simulink model "ASM_Traffic_V2X_Complete_Model_2"  (R2019a)
settings: Solver=ode1  StartTime=SIM.tstart.v  StopTime=Inf  FixedStep=SIM.StepSize.v  RelTol=1e-3
PostLoadFcn:
  | if any(exist('dsrtsu_mdlpostloadfcn', 'file') ~= 0), dsrtsu_mdlpostloadfcn('Execute', bdroot); end
  | try, asm_mdl_postloadfcn(bdroot, 'UpdateModel', 2200); catch, disp(lasterr); end,
undefined symbols (not defined in the file): _SensorPnts_1, _SensorPnts_13, _SensorPnts_17, _SensorPnts_21, _SensorPnts_25, _SensorPnts_29, _SensorPnts_33, _SensorPnts_37, _SensorPnts_41, _SensorPnts_45, _SensorPnts_49, _SensorPnts_5, _SensorPnts_53, _SensorPnts_57, _SensorPnts_9, _to_, CPT, G5A, ITS, MDL, rad, s_to_rpm, SIM
libraries: simulink x169, ASM_VehicleDynamics_lib x126, ASM_Traffic_lib x83, ASM_Utils_lib x49, mdbs x45, ASM_Environment_lib x17, dspindex x12, dsaV2xLibraryAux x10, dsmpblib x6, dsaV2xAsn1Library x4, dsaV2xLibrary x4, ASM_BrakeHydraulics_lib x4
(part 14 of 36)

== system ASM_Traffic_V2X_Complete_Model_2/MDL/VehicleDynamics/Tire/Tire_FR ==
  Coeff_Fric_Road[] : Inport
  " Pos_z_CP_CoorSys_E[m]" : Inport  Port=2
  UnitVec_z_CP_CoorSys_E[x;y;z] : Inport  Port=3
  Pos_Wheels_CoorSys_E[x;y;z][m] : Inport  Port=4
  v_WheelBody_Abs_CoorSys_V[x;y;z][m|s] : Inport  Port=5
  w_Wheel_CoorSys_Abs_V[x;y;z][rad|s] : Inport  Port=6
  RotationMatrix_V_E_T[3x3] : Inport  Port=7
  UnitVec_y_Wheel_CoorSys_V[x;y;z] : Inport  Port=8
  omega_Wheel[rad|s] : Inport  Port=9
  Sw_Tire_Parameter_Set[1|2|3|4] : Inport  Port=10
  Sw_Tire_Model[1TMEasy|2MF] : Inport  Port=11
  Reset[] : Inport  Port=12
  Mode[1Normal|2Mirror] : Inport  Port=13
  p[Pa] : Inport  Port=14
  Bus Selector : BusSelector  OutputSignals=Sw_r_Tire[1:intern;2:extern],r_Tire_extern[m]
  CONTACT_POINT_CALCULATION_FR : ASM_VehicleDynamics_lib/VehicleDynamics/Tire/Tire_FR/CONTACT_POINT_CALCULATION_FR  Tag=ASM_SUBCOMPONENT  ASMProperties=struct('Name','CONTACT_POINT_CALCULATION_FR','Version','6.0','Library','ASM_VehicleDynamics_lib')  ASMInstanceName=contact_point_calculation_fr  ASMInstanceID=1
  Compare To Constant : simulink/Logic and Bit Operations/Compare To Constant  relop===  const=1  OutDataTypeStr=boolean  ZeroCross=off
  Demux : Demux  Outputs=[1 1 1 1 1 1 1]
  EnableMF : simulink/Logic and Bit Operations/Compare To Constant  relop=~=  const=2  OutDataTypeStr=boolean  ZeroCross=off
  IncludedInASMBUS : Terminator
  Multiport Switch : MultiPortSwitch  Inputs=2  SaturateOnIntegerOverflow=on
  Mux : Mux  Inputs=7
  Or : Logic  Operator=OR  AllPortsSameDT=off  OutDataTypeStr=boolean
  TIRE_FORCES_AND_TORQUES_VECTORS_FR : ASM_VehicleDynamics_lib/VehicleDynamics/Tire/Tire_FR/TIRE_FORCES_AND_TORQUES_VECTORS_FR  Tag=ASM_SUBCOMPONENT  ASMProperties=struct('Name','TIRE_FORCES_AND_TORQUES_VECTORS_FR','Version','1.0','Library','ASM_VehicleDynamics_lib')  ASMInstanceName=tire_forces_and_torques_vectors_fr  ASMInstanceID=1
  TIRE_MF : ASM_VehicleDynamics_lib/VehicleDynamics/Tire/TireComponents/TIRE_MF  Tag=ASM_SUBCOMPONENT  Base=MDL.VehicleDynamics.Tire.FR.MF.Base  Para_Set_1=MDL.VehicleDynamics.Tire.FR.MF.Para_Set_1  Para_Set_2=MDL.VehicleDynamics.Tire.FR.MF.Para_Set_2  Para_Set_3=MDL.VehicleDynamics.Tire.FR.MF.Para_Set_3  Para_Set_4=MDL.VehicleDynamics.Tire.FR.MF.Para_Set_4  StepSize=SIM.StepSize  ASMProperties=struct('Name','TIRE_MF','Version','4.0','Library','ASM_VehicleDynamics_lib')  ASMInstanceName=FR  ASMInstanceID=2
      settings: AttributesFormatString=Instance Name: FR\nInstance ID: 2
  TIRE_MODEL_TMEASY_FR : ASM_VehicleDynamics_lib/VehicleDynamics/Tire/Tire_FR/TIRE_MODEL_TMEASY_FR  Tag=ASM_SUBCOMPONENT  Para_Set_1=MDL.VehicleDynamics.Tire.FR.TMEasy.Para_Set_1  Para_Set_2=MDL.VehicleDynamics.Tire.FR.TMEasy.Para_Set_2  Para_Set_3=MDL.VehicleDynamics.Tire.FR.TMEasy.Para_Set_3  Para_Set_4=MDL.VehicleDynamics.Tire.FR.TMEasy.Para_Set_4  StepSize=SIM.StepSize  ASMProperties=struct('Name','TIRE_MODEL_TMEASY_FR','Version','16.0','Library','ASM_VehicleDynamics_lib')  ASMInstanceName=tire_model_tmeasy_fr  ASMInstanceID=1
  F_Tire[x;y;z][N] : Outport
  Trq_Tire[x;y;z][Nm] : Outport  Port=2
  Trq_Tire_Wheel[Nm] : Outport  Port=3
  Stiffness_z_Tire[N|m] : Outport  Port=4
  tag scope: ASMBUS_VehicleDynamics_ContactPoint_FR_Tire=global, ASMBUS_VehicleDynamics_ForcesAndTorques_FR_Tire=global, ASMBUS_VehicleDynamics_MF_FR_Tire=global, ASMBUS_VehicleDynamics_TMEasy_FR_Tire=global
  wires:
  p[Pa]/1 -> TIRE_MF/13
  Mode[1Normal|2Mirror]/1 -> TIRE_MF/12
  Or/1 -> TIRE_MF/9
  EnableMF/1 -> Or/1
  TIRE_MF/2 -> Multiport Switch/3
  Bus Selector/1 -> TIRE_MODEL_TMEASY_FR/10, TIRE_MF/10  "<Sw_r_Tire[1:intern;2:extern]>"
  Bus Selector/2 -> TIRE_MODEL_TMEASY_FR/11, TIRE_MF/11  "<r_Tire_extern[m]>"
  [TAG_Tire_Switches] -> Bus Selector/1
  Multiport Switch/1 -> Demux/1
  Demux/6 -> TIRE_FORCES_AND_TORQUES_VECTORS_FR/6
  Demux/5 -> TIRE_FORCES_AND_TORQUES_VECTORS_FR/5
  Demux/4 -> TIRE_FORCES_AND_TORQUES_VECTORS_FR/4
  Demux/3 -> TIRE_FORCES_AND_TORQUES_VECTORS_FR/3
  Demux/2 -> TIRE_FORCES_AND_TORQUES_VECTORS_FR/2
  Demux/1 -> TIRE_FORCES_AND_TORQUES_VECTORS_FR/1
  Demux/7 -> Stiffness_z_Tire[N|m]/1
  Mux/1 -> Multiport Switch/2
  TIRE_MODEL_TMEASY_FR/8 -> Mux/7
  TIRE_MODEL_TMEASY_FR/7 -> Mux/6
  TIRE_MODEL_TMEASY_FR/6 -> Mux/5
  TIRE_MODEL_TMEASY_FR/5 -> Mux/4
  TIRE_MODEL_TMEASY_FR/4 -> Mux/3
  TIRE_MODEL_TMEASY_FR/3 -> Mux/2
  TIRE_MODEL_TMEASY_FR/2 -> Mux/1
  Reset[]/1 -> Or/2, TIRE_MODEL_TMEASY_FR/9, CONTACT_POINT_CALCULATION_FR/8
  CONTACT_POINT_CALCULATION_FR/11 -> IncludedInASMBUS/1
  CONTACT_POINT_CALCULATION_FR/1 -> [ASMBUS_VehicleDynamics_ContactPoint_FR_Tire]
  TIRE_MF/1 -> [ASMBUS_VehicleDynamics_MF_FR_Tire]
  TIRE_MODEL_TMEASY_FR/1 -> [ASMBUS_VehicleDynamics_TMEasy_FR_Tire]
  Compare To Constant/1 -> TIRE_MODEL_TMEASY_FR/Enable
  RotationMatrix_V_E_T[3x3]/1 -> CONTACT_POINT_CALCULATION_FR/6
  UnitVec_z_CP_CoorSys_E[x;y;z]/1 -> CONTACT_POINT_CALCULATION_FR/5
  " Pos_z_CP_CoorSys_E[m]"/1 -> CONTACT_POINT_CALCULATION_FR/4
  Pos_Wheels_CoorSys_E[x;y;z][m]/1 -> CONTACT_POINT_CALCULATION_FR/3
  w_Wheel_CoorSys_Abs_V[x;y;z][rad|s]/1 -> CONTACT_POINT_CALCULATION_FR/2
  v_WheelBody_Abs_CoorSys_V[x;y;z][m|s]/1 -> CONTACT_POINT_CALCULATION_FR/1
  Sw_Tire_Parameter_Set[1|2|3|4]/1 -> TIRE_MODEL_TMEASY_FR/1, TIRE_MF/1
  TIRE_FORCES_AND_TORQUES_VECTORS_FR/1 -> [ASMBUS_VehicleDynamics_ForcesAndTorques_FR_Tire]
  Coeff_Fric_Road[]/1 -> TIRE_MODEL_TMEASY_FR/2, TIRE_MF/2
  omega_Wheel[rad|s]/1 -> TIRE_MODEL_TMEASY_FR/3, TIRE_MF/3
  UnitVec_y_Wheel_CoorSys_V[x;y;z]/1 -> TIRE_FORCES_AND_TORQUES_VECTORS_FR/11, CONTACT_POINT_CALCULATION_FR/7
  CONTACT_POINT_CALCULATION_FR/2 -> TIRE_MODEL_TMEASY_FR/4, TIRE_MF/4
  CONTACT_POINT_CALCULATION_FR/3 -> TIRE_MODEL_TMEASY_FR/5, TIRE_MF/5
  CONTACT_POINT_CALCULATION_FR/4 -> TIRE_MODEL_TMEASY_FR/6, TIRE_MF/6
  CONTACT_POINT_CALCULATION_FR/5 -> TIRE_MODEL_TMEASY_FR/7, TIRE_MF/7
  CONTACT_POINT_CALCULATION_FR/6 -> TIRE_MODEL_TMEASY_FR/8, TIRE_MF/8
  TIRE_FORCES_AND_TORQUES_VECTORS_FR/2 -> F_Tire[x;y;z][N]/1
  TIRE_FORCES_AND_TORQUES_VECTORS_FR/4 -> Trq_Tire_Wheel[Nm]/1
  TIRE_FORCES_AND_TORQUES_VECTORS_FR/3 -> Trq_Tire[x;y;z][Nm]/1
  CONTACT_POINT_CALCULATION_FR/7 -> TIRE_FORCES_AND_TORQUES_VECTORS_FR/7
  CONTACT_POINT_CALCULATION_FR/8 -> TIRE_FORCES_AND_TORQUES_VECTORS_FR/8
  CONTACT_POINT_CALCULATION_FR/9 -> TIRE_FORCES_AND_TORQUES_VECTORS_FR/9
  CONTACT_POINT_CALCULATION_FR/10 -> TIRE_FORCES_AND_TORQUES_VECTORS_FR/10
  Sw_Tire_Model[1TMEasy|2MF]/1 -> Compare To Constant/1, Multiport Switch/1, EnableMF/1

== system ASM_Traffic_V2X_Complete_Model_2/MDL/VehicleDynamics/Tire/Tire_RL ==
  Coeff_Fric_Road[] : Inport
  " Pos_z_CP_CoorSys_E[m]" : Inport  Port=2
  UnitVec_z_CP_CoorSys_E[x;y;z] : Inport  Port=3
  Pos_Wheels_CoorSys_E[x;y;z][m] : Inport  Port=4
  v_WheelBody_Abs_CoorSys_V[x;y;z][m|s] : Inport  Port=5
  w_Wheel_CoorSys_Abs_V[x;y;z][rad|s] : Inport  Port=6
  RotationMatrix_V_E_T[3x3] : Inport  Port=7
  UnitVec_y_Wheel_CoorSys_V[x;y;z] : Inport  Port=8
  omega_Wheel[rad|s] : Inport  Port=9
  Sw_Tire_Parameter_Set[1|2|3|4] : Inport  Port=10
  Sw_Tire_Model[1TMEasy|2MF] : Inport  Port=11
  Reset[] : Inport  Port=12
  Mode[1Normal|2Mirror] : Inport  Port=13
  p[Pa] : Inport  Port=14
  Bus Selector : BusSelector  OutputSignals=Sw_r_Tire[1:intern;2:extern],r_Tire_extern[m]
  CONTACT_POINT_CALCULATION_RL : ASM_VehicleDynamics_lib/VehicleDynamics/Tire/Tire_RL/CONTACT_POINT_CALCULATION_RL  Tag=ASM_SUBCOMPONENT  ASMProperties=struct('Name','CONTACT_POINT_CALCULATION_RL','Version','6.0','Library','ASM_VehicleDynamics_lib')  ASMInstanceName=contact_point_calculation_rl  ASMInstanceID=1
  Compare To Constant : simulink/Logic and Bit Operations/Compare To Constant  relop===  const=1  OutDataTypeStr=boolean  ZeroCross=off
  Demux : Demux  Outputs=[1 1 1 1 1 1 1]
  EnableMF : simulink/Logic and Bit Operations/Compare To Constant  relop=~=  const=2  OutDataTypeStr=boolean  ZeroCross=off
  IncludedInASMBUS : Terminator
  Multiport Switch : MultiPortSwitch  Inputs=2  SaturateOnIntegerOverflow=on
  Mux : Mux  Inputs=7
  Or : Logic  Operator=OR  AllPortsSameDT=off  OutDataTypeStr=boolean
  TIRE_FORCES_AND_TORQUES_VECTORS_RL : ASM_VehicleDynamics_lib/VehicleDynamics/Tire/Tire_RL/TIRE_FORCES_AND_TORQUES_VECTORS_RL  Tag=ASM_SUBCOMPONENT  ASMProperties=struct('Name','TIRE_FORCES_AND_TORQUES_VECTORS_RL','Version','1.0','Library','ASM_VehicleDynamics_lib')  ASMInstanceName=tire_forces_and_torques_vectors_rl  ASMInstanceID=1
  TIRE_MF : ASM_VehicleDynamics_lib/VehicleDynamics/Tire/TireComponents/TIRE_MF  Tag=ASM_SUBCOMPONENT  Base=MDL.VehicleDynamics.Tire.RL.MF.Base  Para_Set_1=MDL.VehicleDynamics.Tire.RL.MF.Para_Set_1  Para_Set_2=MDL.VehicleDynamics.Tire.RL.MF.Para_Set_2  Para_Set_3=MDL.VehicleDynamics.Tire.RL.MF.Para_Set_3  Para_Set_4=MDL.VehicleDynamics.Tire.RL.MF.Para_Set_4  StepSize=SIM.StepSize  ASMProperties=struct('Name','TIRE_MF','Version','4.0','Library','ASM_VehicleDynamics_lib')  ASMInstanceName=RL  ASMInstanceID=3
      settings: AttributesFormatString=Instance Name: RL\nInstance ID: 3
  TIRE_MODEL_TMEASY_RL : ASM_VehicleDynamics_lib/VehicleDynamics/Tire/Tire_RL/TIRE_MODEL_TMEASY_RL  Tag=ASM_SUBCOMPONENT  Para_Set_1=MDL.VehicleDynamics.Tire.RL.TMEasy.Para_Set_1  Para_Set_2=MDL.VehicleDynamics.Tire.RL.TMEasy.Para_Set_2  Para_Set_3=MDL.VehicleDynamics.Tire.RL.TMEasy.Para_Set_3  Para_Set_4=MDL.VehicleDynamics.Tire.RL.TMEasy.Para_Set_4  StepSize=SIM.StepSize  ASMProperties=struct('Name','TIRE_MODEL_TMEASY_RL','Version','16.0','Library','ASM_VehicleDynamics_lib')  ASMInstanceName=tire_model_tmeasy_rl  ASMInstanceID=1
  F_Tire[x;y;z][N] : Outport
  Trq_Tire[x;y;z][Nm] : Outport  Port=2
  Trq_Tire_Wheel[Nm] : Outport  Port=3
  Stiffness_z_Tire[N|m] : Outport  Port=4
  tag scope: ASMBUS_VehicleDynamics_ContactPoint_RL_Tire=global, ASMBUS_VehicleDynamics_ForcesAndTorques_RL_Tire=global, ASMBUS_VehicleDynamics_MF_RL_Tire=global, ASMBUS_VehicleDynamics_TMEasy_RL_Tire=global
  wires:
  p[Pa]/1 -> TIRE_MF/13
  Mode[1Normal|2Mirror]/1 -> TIRE_MF/12
  Or/1 -> TIRE_MF/9
  EnableMF/1 -> Or/1
  TIRE_MF/2 -> Multiport Switch/3
  Bus Selector/2 -> TIRE_MODEL_TMEASY_RL/11, TIRE_MF/11  "<r_Tire_extern[m]>"
  Bus Selector/1 -> TIRE_MODEL_TMEASY_RL/10, TIRE_MF/10  "<Sw_r_Tire[1:intern;2:extern]>"
  [TAG_Tire_Switches] -> Bus Selector/1
  Multiport Switch/1 -> Demux/1
  Demux/7 -> Stiffness_z_Tire[N|m]/1
  Demux/6 -> TIRE_FORCES_AND_TORQUES_VECTORS_RL/6
  Demux/5 -> TIRE_FORCES_AND_TORQUES_VECTORS_RL/5
  Demux/4 -> TIRE_FORCES_AND_TORQUES_VECTORS_RL/4
  Demux/3 -> TIRE_FORCES_AND_TORQUES_VECTORS_RL/3
  Demux/2 -> TIRE_FORCES_AND_TORQUES_VECTORS_RL/2
  Demux/1 -> TIRE_FORCES_AND_TORQUES_VECTORS_RL/1
  Mux/1 -> Multiport Switch/2
  TIRE_MODEL_TMEASY_RL/8 -> Mux/7
  TIRE_MODEL_TMEASY_RL/7 -> Mux/6
  TIRE_MODEL_TMEASY_RL/6 -> Mux/5
  TIRE_MODEL_TMEASY_RL/5 -> Mux/4
  TIRE_MODEL_TMEASY_RL/4 -> Mux/3
  TIRE_MODEL_TMEASY_RL/3 -> Mux/2
  TIRE_MODEL_TMEASY_RL/2 -> Mux/1
  Reset[]/1 -> TIRE_MODEL_TMEASY_RL/9, Or/2, CONTACT_POINT_CALCULATION_RL/8
  CONTACT_POINT_CALCULATION_RL/11 -> IncludedInASMBUS/1
  TIRE_FORCES_AND_TORQUES_VECTORS_RL/1 -> [ASMBUS_VehicleDynamics_ForcesAndTorques_RL_Tire]
  CONTACT_POINT_CALCULATION_RL/1 -> [ASMBUS_VehicleDynamics_ContactPoint_RL_Tire]
  TIRE_MF/1 -> [ASMBUS_VehicleDynamics_MF_RL_Tire]
  TIRE_MODEL_TMEASY_RL/1 -> [ASMBUS_VehicleDynamics_TMEasy_RL_Tire]
  RotationMatrix_V_E_T[3x3]/1 -> CONTACT_POINT_CALCULATION_RL/6
  UnitVec_z_CP_CoorSys_E[x;y;z]/1 -> CONTACT_POINT_CALCULATION_RL/5
  " Pos_z_CP_CoorSys_E[m]"/1 -> CONTACT_POINT_CALCULATION_RL/4
  Pos_Wheels_CoorSys_E[x;y;z][m]/1 -> CONTACT_POINT_CALCULATION_RL/3
  w_Wheel_CoorSys_Abs_V[x;y;z][rad|s]/1 -> CONTACT_POINT_CALCULATION_RL/2
  v_WheelBody_Abs_CoorSys_V[x;y;z][m|s]/1 -> CONTACT_POINT_CALCULATION_RL/1
  Compare To Constant/1 -> TIRE_MODEL_TMEASY_RL/Enable
  Sw_Tire_Model[1TMEasy|2MF]/1 -> Compare To Constant/1, Multiport Switch/1, EnableMF/1
  CONTACT_POINT_CALCULATION_RL/10 -> TIRE_FORCES_AND_TORQUES_VECTORS_RL/10
  CONTACT_POINT_CALCULATION_RL/9 -> TIRE_FORCES_AND_TORQUES_VECTORS_RL/9
  CONTACT_POINT_CALCULATION_RL/8 -> TIRE_FORCES_AND_TORQUES_VECTORS_RL/8
  CONTACT_POINT_CALCULATION_RL/7 -> TIRE_FORCES_AND_TORQUES_VECTORS_RL/7
  TIRE_FORCES_AND_TORQUES_VECTORS_RL/3 -> Trq_Tire[x;y;z][Nm]/1
  TIRE_FORCES_AND_TORQUES_VECTORS_RL/4 -> Trq_Tire_Wheel[Nm]/1
  TIRE_FORCES_AND_TORQUES_VECTORS_RL/2 -> F_Tire[x;y;z][N]/1
  CONTACT_POINT_CALCULATION_RL/6 -> TIRE_MODEL_TMEASY_RL/8, TIRE_MF/8
  CONTACT_POINT_CALCULATION_RL/5 -> TIRE_MODEL_TMEASY_RL/7, TIRE_MF/7
  CONTACT_POINT_CALCULATION_RL/4 -> TIRE_MODEL_TMEASY_RL/6, TIRE_MF/6
  CONTACT_POINT_CALCULATION_RL/3 -> TIRE_MODEL_TMEASY_RL/5, TIRE_MF/5
  CONTACT_POINT_CALCULATION_RL/2 -> TIRE_MODEL_TMEASY_RL/4, TIRE_MF/4
  UnitVec_y_Wheel_CoorSys_V[x;y;z]/1 -> TIRE_FORCES_AND_TORQUES_VECTORS_RL/11, CONTACT_POINT_CALCULATION_RL/7
  omega_Wheel[rad|s]/1 -> TIRE_MODEL_TMEASY_RL/3, TIRE_MF/3
  Coeff_Fric_Road[]/1 -> TIRE_MODEL_TMEASY_RL/2, TIRE_MF/2
  Sw_Tire_Parameter_Set[1|2|3|4]/1 -> TIRE_MODEL_TMEASY_RL/1, TIRE_MF/1

== system ASM_Traffic_V2X_Complete_Model_2/MDL/VehicleDynamics/Tire/Tire_RR ==
  Coeff_Fric_Road[] : Inport
  " Pos_z_CP_CoorSys_E[m]" : Inport  Port=2
  UnitVec_z_CP_CoorSys_E[x;y;z] : Inport  Port=3
  Pos_Wheels_CoorSys_E[x;y;z][m] : Inport  Port=4
  v_WheelBody_Abs_CoorSys_V[x;y;z][m|s] : Inport  Port=5
  w_Wheel_CoorSys_Abs_V[x;y;z][rad|s] : Inport  Port=6
  RotationMatrix_V_E_T[3x3] : Inport  Port=7
  UnitVec_y_Wheel_CoorSys_V[x;y;z] : Inport  Port=8
  omega_Wheel[rad|s] : Inport  Port=9
  Sw_Tire_Parameter_Set[1|2|3|4] : Inport  Port=10
  Sw_Tire_Model[1TMEasy|2MF] : Inport  Port=11
  Reset[] : Inport  Port=12
  Mode[1Normal|2Mirror] : Inport  Port=13
  p[Pa] : Inport  Port=14
  Bus Selector : BusSelector  OutputSignals=Sw_r_Tire[1:intern;2:extern],r_Tire_extern[m]
  CONTACT_POINT_CALCULATION_RR : ASM_VehicleDynamics_lib/VehicleDynamics/Tire/Tire_RR/CONTACT_POINT_CALCULATION_RR  Tag=ASM_SUBCOMPONENT  ASMProperties=struct('Name','CONTACT_POINT_CALCULATION_RR','Version','6.0','Library','ASM_VehicleDynamics_lib')  ASMInstanceName=contact_point_calculation_rr  ASMInstanceID=1
  Compare To Constant : simulink/Logic and Bit Operations/Compare To Constant  relop===  const=1  OutDataTypeStr=boolean  ZeroCross=off
  Demux : Demux  Outputs=[1 1 1 1 1 1 1]
  EnableMF : simulink/Logic and Bit Operations/Compare To Constant  relop=~=  const=2  OutDataTypeStr=boolean  ZeroCross=off
  IncludedInASMBUS : Terminator
  Multiport Switch : MultiPortSwitch  Inputs=2  SaturateOnIntegerOverflow=on
  Mux : Mux  Inputs=7
  Or : Logic  Operator=OR  AllPortsSameDT=off  OutDataTypeStr=boolean
  TIRE_FORCES_AND_TORQUES_VECTORS_RR : ASM_VehicleDynamics_lib/VehicleDynamics/Tire/Tire_RR/TIRE_FORCES_AND_TORQUES_VECTORS_RR  Tag=ASM_SUBCOMPONENT  ASMProperties=struct('Name','TIRE_FORCES_AND_TORQUES_VECTORS_RR','Version','1.0','Library','ASM_VehicleDynamics_lib')  ASMInstanceName=tire_forces_and_torques_vectors_rr  ASMInstanceID=1
  TIRE_MF : ASM_VehicleDynamics_lib/VehicleDynamics/Tire/TireComponents/TIRE_MF  Tag=ASM_SUBCOMPONENT  Base=MDL.VehicleDynamics.Tire.RR.MF.Base  Para_Set_1=MDL.VehicleDynamics.Tire.RR.MF.Para_Set_1  Para_Set_2=MDL.VehicleDynamics.Tire.RR.MF.Para_Set_2  Para_Set_3=MDL.VehicleDynamics.Tire.RR.MF.Para_Set_3  Para_Set_4=MDL.VehicleDynamics.Tire.RR.MF.Para_Set_4  StepSize=SIM.StepSize  ASMProperties=struct('Name','TIRE_MF','Version','4.0','Library','ASM_VehicleDynamics_lib')  ASMInstanceName=RR  ASMInstanceID=4
      settings: AttributesFormatString=Instance Name: RR\nInstance ID: 4
  TIRE_MODEL_TMEASY_RR : ASM_VehicleDynamics_lib/VehicleDynamics/Tire/Tire_RR/TIRE_MODEL_TMEASY_RR  Tag=ASM_SUBCOMPONENT  Para_Set_1=MDL.VehicleDynamics.Tire.RR.TMEasy.Para_Set_1  Para_Set_2=MDL.VehicleDynamics.Tire.RR.TMEasy.Para_Set_2  Para_Set_3=MDL.VehicleDynamics.Tire.RR.TMEasy.Para_Set_3  Para_Set_4=MDL.VehicleDynamics.Tire.RR.TMEasy.Para_Set_4  StepSize=SIM.StepSize  ASMProperties=struct('Name','TIRE_MODEL_TMEASY_RR','Version','16.0','Library','ASM_VehicleDynamics_lib')  ASMInstanceName=tire_model_tmeasy_rr  ASMInstanceID=1
  F_Tire[x;y;z][N] : Outport
  Trq_Tire[x;y;z][Nm] : Outport  Port=2
  Trq_Tire_Wheel[Nm] : Outport  Port=3
  Stiffness_z_Tire[N|m] : Outport  Port=4
  tag scope: ASMBUS_VehicleDynamics_ContactPoint_RR_Tire=global, ASMBUS_VehicleDynamics_ForcesAndTorques_RR_Tire=global, ASMBUS_VehicleDynamics_MF_RR_Tire=global, ASMBUS_VehicleDynamics_TMEasy_RR_Tire=global
  wires:
  p[Pa]/1 -> TIRE_MF/13
  Mode[1Normal|2Mirror]/1 -> TIRE_MF/12
  Or/1 -> TIRE_MF/9
  EnableMF/1 -> Or/1
  TIRE_MF/2 -> Multiport Switch/3
  Bus Selector/2 -> TIRE_MODEL_TMEASY_RR/11, TIRE_MF/11  "<r_Tire_extern[m]>"
  Bus Selector/1 -> TIRE_MODEL_TMEASY_RR/10, TIRE_MF/10  "<Sw_r_Tire[1:intern;2:extern]>"
  [TAG_Tire_Switches] -> Bus Selector/1
  Multiport Switch/1 -> Demux/1
  Demux/7 -> Stiffness_z_Tire[N|m]/1
  Demux/6 -> TIRE_FORCES_AND_TORQUES_VECTORS_RR/6
  Demux/5 -> TIRE_FORCES_AND_TORQUES_VECTORS_RR/5
  Demux/4 -> TIRE_FORCES_AND_TORQUES_VECTORS_RR/4
  Demux/3 -> TIRE_FORCES_AND_TORQUES_VECTORS_RR/3
  Demux/2 -> TIRE_FORCES_AND_TORQUES_VECTORS_RR/2
  Demux/1 -> TIRE_FORCES_AND_TORQUES_VECTORS_RR/1
  Mux/1 -> Multiport Switch/2
  TIRE_MODEL_TMEASY_RR/8 -> Mux/7
  TIRE_MODEL_TMEASY_RR/7 -> Mux/6
  TIRE_MODEL_TMEASY_RR/6 -> Mux/5
  TIRE_MODEL_TMEASY_RR/5 -> Mux/4
  TIRE_MODEL_TMEASY_RR/4 -> Mux/3
  TIRE_MODEL_TMEASY_RR/3 -> Mux/2
  TIRE_MODEL_TMEASY_RR/2 -> Mux/1
  Reset[]/1 -> Or/2, TIRE_MODEL_TMEASY_RR/9, CONTACT_POINT_CALCULATION_RR/8
  CONTACT_POINT_CALCULATION_RR/11 -> IncludedInASMBUS/1
  TIRE_FORCES_AND_TORQUES_VECTORS_RR/1 -> [ASMBUS_VehicleDynamics_ForcesAndTorques_RR_Tire]
  CONTACT_POINT_CALCULATION_RR/1 -> [ASMBUS_VehicleDynamics_ContactPoint_RR_Tire]
  TIRE_MF/1 -> [ASMBUS_VehicleDynamics_MF_RR_Tire]
  TIRE_MODEL_TMEASY_RR/1 -> [ASMBUS_VehicleDynamics_TMEasy_RR_Tire]
  RotationMatrix_V_E_T[3x3]/1 -> CONTACT_POINT_CALCULATION_RR/6
  UnitVec_z_CP_CoorSys_E[x;y;z]/1 -> CONTACT_POINT_CALCULATION_RR/5
  " Pos_z_CP_CoorSys_E[m]"/1 -> CONTACT_POINT_CALCULATION_RR/4
  Pos_Wheels_CoorSys_E[x;y;z][m]/1 -> CONTACT_POINT_CALCULATION_RR/3
  w_Wheel_CoorSys_Abs_V[x;y;z][rad|s]/1 -> CONTACT_POINT_CALCULATION_RR/2
  v_WheelBody_Abs_CoorSys_V[x;y;z][m|s]/1 -> CONTACT_POINT_CALCULATION_RR/1
  Sw_Tire_Parameter_Set[1|2|3|4]/1 -> TIRE_MODEL_TMEASY_RR/1, TIRE_MF/1
  Coeff_Fric_Road[]/1 -> TIRE_MODEL_TMEASY_RR/2, TIRE_MF/2
  omega_Wheel[rad|s]/1 -> TIRE_MODEL_TMEASY_RR/3, TIRE_MF/3
  UnitVec_y_Wheel_CoorSys_V[x;y;z]/1 -> TIRE_FORCES_AND_TORQUES_VECTORS_RR/11, CONTACT_POINT_CALCULATION_RR/7
  CONTACT_POINT_CALCULATION_RR/2 -> TIRE_MODEL_TMEASY_RR/4, TIRE_MF/4
  CONTACT_POINT_CALCULATION_RR/3 -> TIRE_MODEL_TMEASY_RR/5, TIRE_MF/5
  CONTACT_POINT_CALCULATION_RR/4 -> TIRE_MODEL_TMEASY_RR/6, TIRE_MF/6
  CONTACT_POINT_CALCULATION_RR/5 -> TIRE_MODEL_TMEASY_RR/7, TIRE_MF/7
  CONTACT_POINT_CALCULATION_RR/6 -> TIRE_MODEL_TMEASY_RR/8, TIRE_MF/8
  TIRE_FORCES_AND_TORQUES_VECTORS_RR/2 -> F_Tire[x;y;z][N]/1
  TIRE_FORCES_AND_TORQUES_VECTORS_RR/4 -> Trq_Tire_Wheel[Nm]/1
  TIRE_FORCES_AND_TORQUES_VECTORS_RR/3 -> Trq_Tire[x;y;z][Nm]/1
  CONTACT_POINT_CALCULATION_RR/7 -> TIRE_FORCES_AND_TORQUES_VECTORS_RR/7
  CONTACT_POINT_CALCULATION_RR/8 -> TIRE_FORCES_AND_TORQUES_VECTORS_RR/8
  CONTACT_POINT_CALCULATION_RR/9 -> TIRE_FORCES_AND_TORQUES_VECTORS_RR/9
  CONTACT_POINT_CALCULATION_RR/10 -> TIRE_FORCES_AND_TORQUES_VECTORS_RR/10
  Sw_Tire_Model[1TMEasy|2MF]/1 -> Compare To Constant/1, EnableMF/1, Multiport Switch/1
  Compare To Constant/1 -> TIRE_MODEL_TMEASY_RR/Enable

== system ASM_Traffic_V2X_Complete_Model_2/MDL/VehicleDynamics/VehicleMovement/ASMSignalCollector ==
  Reset[] : Inport
  VEHICLE_MOVEMENT_INFO_CAR : ASM_VehicleDynamics_lib/VehicleDynamics/VehicleMovement/VEHICLE_MOVEMENT_INFO_CAR  StepSize=SIM.StepSize  ASMProperties=struct('Name','VEHICLE_MOVEMENT_INFO_CAR','Version','10.0','Library','ASM_VehicleDynamics_lib')
  ASMSignalBus : Outport
  wires:
  [ASMBUS_VehicleDynamics_Steering] -> VEHICLE_MOVEMENT_INFO_CAR/9
  VEHICLE_MOVEMENT_INFO_CAR/1 -> ASMSignalBus/1
  [ASMBUS_VehicleDynamics_Suspension] -> VEHICLE_MOVEMENT_INFO_CAR/8
  [ASMBUS_VehicleDynamics_SensorMotion] -> VEHICLE_MOVEMENT_INFO_CAR/7
  [ASMBUS_VehicleDynamics_VehicleMass] -> VEHICLE_MOVEMENT_INFO_CAR/6
  [ASMBUS_VehicleDynamics_MassForcesAndTorques] -> VEHICLE_MOVEMENT_INFO_CAR/5
  Reset[]/1 -> VEHICLE_MOVEMENT_INFO_CAR/1
  [ASMBUS_VehicleDynamics_CoordinateTransformation] -> VEHICLE_MOVEMENT_INFO_CAR/3
  [ASMBUS_VehicleDynamics_CoGAndWheelVelocities] -> VEHICLE_MOVEMENT_INFO_CAR/2
  [ASMBUS_VehicleDynamics_VehicleMotion] -> VEHICLE_MOVEMENT_INFO_CAR/4

== system ASM_Traffic_V2X_Complete_Model_2/MDL/VehicleDynamics/VehicleMovement/OR ==
  In1 : Inport
  In2 : Inport  Port=2
  Data Type Conversion : DataTypeConversion  OutDataTypeStr=double
  Logical Operator : Logic  Operator=OR  AllPortsSameDT=off
  Out : Outport
  wires:
  Data Type Conversion/1 -> Out/1
  In2/1 -> Logical Operator/2
  In1/1 -> Logical Operator/1
  Logical Operator/1 -> Data Type Conversion/1

== system ASM_Traffic_V2X_Complete_Model_2/MDLUserInterface/Drivetrain/MDL_DISP/ActiveTransmission ==
  ActiveTrm : Inport
  ActiveTransmission : Scope  NumInputPorts=6
  Bus Selector : BusSelector  OutputSignals=omega_In_Trm[rad|s],omega_Out_Trm[rad|s],Trq_Out_Trm[Nm],i_Trm[],Inertia_Trm[kgm2],i_unsync_Trm[]
  Inertia_Trm[kgm2] : Subsystem
      mask Display: disp('')
  Trq_Out_Trm[Nm] : Subsystem
      mask Display: disp('')
  i_Trm[] : Subsystem
      mask Display: disp('')
  i_unsync_Trm[] : Subsystem
      mask Display: disp('')
  omega_In_Trm[rad|s] : Subsystem
      mask Display: disp('')
  omega_Out_Trm[rad|s] : Subsystem
      mask Display: disp('')
  wires:
  ActiveTrm/1 -> Bus Selector/1
  Bus Selector/1 -> omega_In_Trm[rad|s]/1(In1)  "<omega_In_Trm[rad|s]>"
  omega_In_Trm[rad|s]/1(Out1) -> ActiveTransmission/1  "omega_In_Trm[rad|s]"
  Bus Selector/2 -> omega_Out_Trm[rad|s]/1(In1)  "<omega_Out_Trm[rad|s]>"
  omega_Out_Trm[rad|s]/1(Out1) -> ActiveTransmission/2  "omega_Out_Trm[rad|s]"
  Bus Selector/3 -> Trq_Out_Trm[Nm]/1(In1)  "<Trq_Out_Trm[Nm]>"
  Trq_Out_Trm[Nm]/1(Out1) -> ActiveTransmission/3  "Trq_Out_Trm[Nm]"
  Bus Selector/4 -> i_Trm[]/1(In1)  "<i_Trm[]>"
  i_Trm[]/1(Out1) -> ActiveTransmission/4  "i_Trm[]"
  Bus Selector/5 -> Inertia_Trm[kgm2]/1(In1)  "<Inertia_Trm[kgm2]>"
  Inertia_Trm[kgm2]/1(Out1) -> ActiveTransmission/5  "Inertia_Trm[kgm2]"
  Bus Selector/6 -> i_unsync_Trm[]/1(In1)  "<i_unsync_Trm[]>"
  i_unsync_Trm[]/1(Out1) -> ActiveTransmission/6  "i_unsync_Trm[]"

== system ASM_Traffic_V2X_Complete_Model_2/MDLUserInterface/Drivetrain/MDL_DISP/AutomaticTransmission ==
  AutoTrm : Inport
  Bus Selector : BusSelector  OutputSignals=LockUpClutch.Trq_Fric_Clutch[Nm],LockUpClutch.Trq_TorsionSpring_Clutch[Nm],LockUpClutch.omega_Out_ClutchPlate[rad|s],TorqueConverter.Trq_Turbine[Nm],TorqueConverter.Trq_Pump[Nm]
  LookUpClutch : Scope  NumInputPorts=3
  TorqueConverter : Scope  NumInputPorts=2
  Trq_Fric_Clutch[Nm] : Subsystem
      mask Display: disp('')
  Trq_Pump[Nm] : Subsystem
      mask Display: disp('')
  Trq_TorsionSpring_Clutch[Nm] : Subsystem
      mask Display: disp('')
  Trq_Turbine[Nm] : Subsystem
      mask Display: disp('')
  omega_Out_ClutchPlate[rad|s] : Subsystem
      mask Display: disp('')
  wires:
  AutoTrm/1 -> Bus Selector/1
  Trq_Fric_Clutch[Nm]/1(Out1) -> LookUpClutch/1  "Trq_Fric_Clutch[Nm]"
  Trq_TorsionSpring_Clutch[Nm]/1(Out1) -> LookUpClutch/2  "Trq_TorsionSpring_Clutch[Nm]"
  omega_Out_ClutchPlate[rad|s]/1(Out1) -> LookUpClutch/3  "omega_Out_ClutchPlate[rad|s]"
  Trq_Turbine[Nm]/1(Out1) -> TorqueConverter/1  "Trq_Turbine[Nm]"
  Trq_Pump[Nm]/1(Out1) -> TorqueConverter/2  "Trq_Pump[Nm]"
  Bus Selector/1 -> Trq_Fric_Clutch[Nm]/1(In1)  "<Trq_Fric_Clutch[Nm]>"
  Bus Selector/2 -> Trq_TorsionSpring_Clutch[Nm]/1(In1)  "<Trq_TorsionSpring_Clutch[Nm]>"
  Bus Selector/3 -> omega_Out_ClutchPlate[rad|s]/1(In1)  "<omega_Out_ClutchPlate[rad|s]>"
  Bus Selector/4 -> Trq_Turbine[Nm]/1(In1)  "<Trq_Turbine[Nm]>"
  Bus Selector/5 -> Trq_Pump[Nm]/1(In1)  "<Trq_Pump[Nm]>"

== system ASM_Traffic_V2X_Complete_Model_2/MDLUserInterface/Drivetrain/MDL_DISP/EngineSpeed ==
  Crankshaft : Inport
  Starter : Inport  Port=2
  Bus Selector : BusSelector  OutputSignals=n_Engine[rpm]
  Bus Selector1 : BusSelector  OutputSignals=Trq_Starter[Nm]
  EngineSpeed : Scope  NumInputPorts=2
  Trq_Starter[Nm] : Subsystem
      mask Display: disp('')
  n_Engine[rpm] : Subsystem
      mask Display: disp('')
  wires:
  Crankshaft/1 -> Bus Selector/1
  Bus Selector/1 -> n_Engine[rpm]/1(In1)  "<n_Engine[rpm]>"
  n_Engine[rpm]/1(Out1) -> EngineSpeed/1  "n_Engine[rpm]"
  Bus Selector1/1 -> Trq_Starter[Nm]/1(In1)  "<Trq_Starter[Nm]>"
  Trq_Starter[Nm]/1(Out1) -> EngineSpeed/2  "Trq_Starter[Nm]"
  Starter/1 -> Bus Selector1/1

== system ASM_Traffic_V2X_Complete_Model_2/MDLUserInterface/Drivetrain/MDL_DISP/ManualTransmission ==
  ManTrm : Inport
  Bus Selector : BusSelector  OutputSignals=Clutch.Trq_Fric_Clutch[Nm],Clutch.Trq_TorsionSpring_Clutch[Nm],Clutch.omega_Out_ClutchPlate[rad|s]
  Clutch : Scope  NumInputPorts=3
  Trq_Fric_Clutch[Nm] : Subsystem
      mask Display: disp('')
  Trq_TorsionSpring_Clutch[Nm] : Subsystem
      mask Display: disp('')
  omega_Out_ClutchPlate[rad|s] : Subsystem
      mask Display: disp('')
  wires:
  ManTrm/1 -> Bus Selector/1
  Trq_Fric_Clutch[Nm]/1(Out1) -> Clutch/1  "Trq_Fric_Clutch[Nm]"
  Trq_TorsionSpring_Clutch[Nm]/1(Out1) -> Clutch/2  "Trq_TorsionSpring_Clutch[Nm]"
  omega_Out_ClutchPlate[rad|s]/1(Out1) -> Clutch/3  "omega_Out_ClutchPlate[rad|s]"
  Bus Selector/1 -> Trq_Fric_Clutch[Nm]/1(In1)  "<Trq_Fric_Clutch[Nm]>"
  Bus Selector/2 -> Trq_TorsionSpring_Clutch[Nm]/1(In1)  "<Trq_TorsionSpring_Clutch[Nm]>"
  Bus Selector/3 -> omega_Out_ClutchPlate[rad|s]/1(In1)  "<omega_Out_ClutchPlate[rad|s]>"

== system ASM_Traffic_V2X_Complete_Model_2/MDLUserInterface/Drivetrain/MDL_DISP/Shafts ==
  Shaft_CF : Inport
  Shaft_CR : Inport  Port=2
  Shaft_FL : Inport  Port=3
  Shaft_FR : Inport  Port=4
  Shaft_RL : Inport  Port=5
  Shaft_RR : Inport  Port=6
  Bus Selector : BusSelector  OutputSignals=Trq_CF_Shaft[Nm]
  Bus Selector1 : BusSelector  OutputSignals=Trq_CR_Shaft[Nm]
  Bus Selector2 : BusSelector  OutputSignals=Trq_FL_Shaft[Nm]
  Bus Selector3 : BusSelector  OutputSignals=Trq_FR_Shaft[Nm]
  Bus Selector4 : BusSelector  OutputSignals=Trq_RL_Shaft[Nm]
  Bus Selector5 : BusSelector  OutputSignals=Trq_RR_Shaft[Nm]
  Shafts : Scope  NumInputPorts=6
  Trq_CF_Shaft[Nm] : Subsystem
      mask Display: disp('')
  Trq_CR_Shaft[Nm] : Subsystem
      mask Display: disp('')
  Trq_FL_Shaft[Nm] : Subsystem
      mask Display: disp('')
  Trq_FR_Shaft[Nm] : Subsystem
      mask Display: disp('')
  Trq_RL_Shaft[Nm] : Subsystem
      mask Display: disp('')
  Trq_RR_Shaft[Nm] : Subsystem
      mask Display: disp('')
  wires:
  Bus Selector/1 -> Trq_CF_Shaft[Nm]/1(In1)  "<Trq_CF_Shaft[Nm]>"
  Trq_CF_Shaft[Nm]/1(Out1) -> Shafts/1  "Trq_CF_Shaft[Nm]"
  Bus Selector1/1 -> Trq_CR_Shaft[Nm]/1(In1)  "<Trq_CR_Shaft[Nm]>"
  Trq_CR_Shaft[Nm]/1(Out1) -> Shafts/2  "Trq_CR_Shaft[Nm]"
  Bus Selector2/1 -> Trq_FL_Shaft[Nm]/1(In1)  "<Trq_FL_Shaft[Nm]>"
  Trq_FL_Shaft[Nm]/1(Out1) -> Shafts/3  "Trq_FL_Shaft[Nm]"
  Bus Selector3/1 -> Trq_FR_Shaft[Nm]/1(In1)  "<Trq_FR_Shaft[Nm]>"
  Trq_FR_Shaft[Nm]/1(Out1) -> Shafts/4  "Trq_FR_Shaft[Nm]"
  Bus Selector4/1 -> Trq_RL_Shaft[Nm]/1(In1)  "<Trq_RL_Shaft[Nm]>"
  Trq_RL_Shaft[Nm]/1(Out1) -> Shafts/5  "Trq_RL_Shaft[Nm]"
  Bus Selector5/1 -> Trq_RR_Shaft[Nm]/1(In1)  "<Trq_RR_Shaft[Nm]>"
  Trq_RR_Shaft[Nm]/1(Out1) -> Shafts/6  "Trq_RR_Shaft[Nm]"
  Shaft_CF/1 -> Bus Selector/1
  Shaft_CR/1 -> Bus Selector1/1
  Shaft_FL/1 -> Bus Selector2/1
  Shaft_FR/1 -> Bus Selector3/1
  Shaft_RL/1 -> Bus Selector4/1
  Shaft_RR/1 -> Bus Selector5/1

== system ASM_Traffic_V2X_Complete_Model_2/MDLUserInterface/Engine/MDL_DISP/CO2_Emission[kg|100km] ==
  In1 : Inport
  Out1 : Outport
  wires:
  In1/1 -> Out1/1

== system ASM_Traffic_V2X_Complete_Model_2/MDLUserInterface/Engine/MDL_DISP/CO2_Emission[kg|100km]_ ==
  v_Vehicle[km|h] : Inport
  CO2_Emission[kg|h] : Inport  Port=2
  Product : Product  Inputs=*/  SaturateOnIntegerOverflow=on  OutDataTypeStr=Inherit: Same as first input
  Saturation : Saturate  UpperLimit=inf  LowerLimit=eps
  Saturation1 : Saturate  UpperLimit=1000  LowerLimit=0
  "[kg|km]2[kg|100km]" : Gain  Gain=100  SaturateOnIntegerOverflow=on  OutDataTypeStr=Inherit: Same as input  ParamDataTypeStr=Inherit: Same as input
  CO2_Emission[kg|100km] : Outport
  wires:
  CO2_Emission[kg|h]/1 -> Product/1
  Saturation/1 -> Product/2
  Product/1 -> "[kg|km]2[kg|100km]"/1
  "[kg|km]2[kg|100km]"/1 -> Saturation1/1
  v_Vehicle[km|h]/1 -> Saturation/1
  Saturation1/1 -> CO2_Emission[kg|100km]/1

== system ASM_Traffic_V2X_Complete_Model_2/MDLUserInterface/Engine/MDL_DISP/CO2_Emission[kg|h] ==
  In1 : Inport
  Out1 : Outport
  wires:
  In1/1 -> Out1/1

== system ASM_Traffic_V2X_Complete_Model_2/MDLUserInterface/Engine/MDL_DISP/CO2_Emission_Total[kg] ==
  In1 : Inport
  Out1 : Outport
  wires:
  In1/1 -> Out1/1

== system ASM_Traffic_V2X_Complete_Model_2/MDLUserInterface/Engine/MDL_DISP/FuelTank[0|1] ==
  In1 : Inport
  Out1 : Outport
  wires:
  In1/1 -> Out1/1

== system ASM_Traffic_V2X_Complete_Model_2/MDLUserInterface/Engine/MDL_DISP/Fuel_Consumption[L|100km] ==
  In1 : Inport
  Out1 : Outport
  wires:
  In1/1 -> Out1/1

== system ASM_Traffic_V2X_Complete_Model_2/MDLUserInterface/Engine/MDL_DISP/Fuel_Consumption[L|100km]_ ==
  v_Vehicle[km|h] : Inport
  Fuel_Consumption[l|h] : Inport  Port=2
  Product : Product  Inputs=*/  SaturateOnIntegerOverflow=on  OutDataTypeStr=Inherit: Same as first input
  Saturation : Saturate  UpperLimit=inf  LowerLimit=eps
  Saturation1 : Saturate  UpperLimit=1000  LowerLimit=0
  "[l|km]2[l|100km]" : Gain  Gain=100  SaturateOnIntegerOverflow=on  OutDataTypeStr=Inherit: Same as input  ParamDataTypeStr=Inherit: Same as input
  Fuel_Consumption[l|100km] : Outport
  wires:
  Saturation1/1 -> Fuel_Consumption[l|100km]/1
  v_Vehicle[km|h]/1 -> Saturation/1
  "[l|km]2[l|100km]"/1 -> Saturation1/1
  Product/1 -> "[l|km]2[l|100km]"/1
  Saturation/1 -> Product/2
  Fuel_Consumption[l|h]/1 -> Product/1

== system ASM_Traffic_V2X_Complete_Model_2/MDLUserInterface/Engine/MDL_DISP/Fuel_Consumption[l|h] ==
  In1 : Inport
  Out1 : Outport
  wires:
  In1/1 -> Out1/1

== system ASM_Traffic_V2X_Complete_Model_2/MDLUserInterface/Engine/MDL_DISP/Fuel_Consumption_Total[l] ==
  In1 : Inport
  Out1 : Outport
  wires:
  In1/1 -> Out1/1

== system ASM_Traffic_V2X_Complete_Model_2/MDLUserInterface/Engine/MDL_DISP/T_Water[degC] ==
  In1 : Inport
  Out1 : Outport
  wires:
  In1/1 -> Out1/1

== system ASM_Traffic_V2X_Complete_Model_2/MDLUserInterface/Engine/MDL_DISP/Trq_Eff_Engine[Nm] ==
  In1 : Inport
  Out1 : Outport
  wires:
  In1/1 -> Out1/1

== system ASM_Traffic_V2X_Complete_Model_2/MDLUserInterface/Engine/MDL_DISP/Trq_Fric_Engine[Nm] ==
  In1 : Inport
  Out1 : Outport
  wires:
  In1/1 -> Out1/1

== system ASM_Traffic_V2X_Complete_Model_2/MDLUserInterface/Engine/MDL_DISP/Trq_Ind_Engine[Nm] ==
  In1 : Inport
  Out1 : Outport
  wires:
  In1/1 -> Out1/1

== system ASM_Traffic_V2X_Complete_Model_2/MDLUserInterface/Engine/MDL_DISP/b_e[g|kWh] ==
  In1 : Inport
  Out1 : Outport
  wires:
  In1/1 -> Out1/1

== system ASM_Traffic_V2X_Complete_Model_2/MDLUserInterface/Engine/MDL_DISP/eta_Eff_Engine[0_1] ==
  In1 : Inport
  Out1 : Outport
  wires:
  In1/1 -> Out1/1

== system ASM_Traffic_V2X_Complete_Model_2/MDLUserInterface/Engine/MDL_DISP/eta_Ind_Engine[0_1] ==
  In1 : Inport
  Out1 : Outport
  wires:
  In1/1 -> Out1/1

== system ASM_Traffic_V2X_Complete_Model_2/MDLUserInterface/Engine/MDL_DISP/eta_Mechanical_Engine[0_1] ==
  In1 : Inport
  Out1 : Outport
  wires:
  In1/1 -> Out1/1

== system ASM_Traffic_V2X_Complete_Model_2/MDLUserInterface/Engine/MDL_DISP/mdot_Fuel[g|h] ==
  In1 : Inport
  Out1 : Outport
  wires:
  In1/1 -> Out1/1

== system ASM_Traffic_V2X_Complete_Model_2/MDLUserInterface/Environment/MDL_DISP/Driver ==
  Driver : Inport
  Velocities : Inport  Port=2
  AbsoluteError : Subsystem
  Angle_SteeringWheel[deg] : Subsystem
      mask Display: disp('')
  Bus Selector1 : BusSelector  OutputSignals=Vehicle.Linear.v_Vehicle_CoG[x;y;z][km|h].v_x_Vehicle_CoG[km|h]
  Bus Selector2 : BusSelector  OutputSignals=ReferenceVelocity.v_Vehicle_Ref[km|h],OutputSignals.Pos_AccPedal[%],OutputSignals.Pos_BrakePedal[%],OutputSignals.Pos_ClutchPedal[%],OutputSignals.Gear[],OutputSignals.AutomaticTrmCtrlSignals.SelectorLever[-3T|-2P|-1R|0N|1D]
  Bus Selector3 : BusSelector  OutputSignals=ReferenceVelocity.a_x_Vehicle_Ref[m|s2],OutputSignals.Angle_SteeringWheel[deg],LateralController.PositionError.e_Lat[m]
  DriverOverview : Scope  NumInputPorts=8
  Gear[] : Subsystem
      mask Display: disp('')
  Mux : Mux  Inputs=3
  Mux1 : Mux  Inputs=2
  Mux2 : Mux  Inputs=2
  Pos_AccPedal[%] : Subsystem
      mask Display: disp('')
  Pos_BrakePedal[%] : Subsystem
      mask Display: disp('')
  Pos_ClutchPedal[%] : Subsystem
      mask Display: disp('')
  RelativeError : Subsystem  mask{UpLim=100, LowLim=-100}
      mask prompts: UpLim "Upper Limit"; LowLim "Lower Limit"
  SelectorLever[-3T|-2P|-1R|0N|1D] : Subsystem
      mask Display: disp('')
  a_x_Vehicle_Ref[m|s2] : Subsystem
      mask Display: disp('')
  e_Lat[m] : Subsystem
      mask Display: disp('')
  v_Vehicle_Ref[km|h] : Subsystem
      mask Display: disp('')
  v_x_Vehicle_CoG[km|h] : Subsystem
      mask Display: disp('')
  wires:
  Driver/1 -> Bus Selector3/1, Bus Selector2/1
  Pos_AccPedal[%]/1(Out1) -> Mux/1  "Pos_AccPedal[%]"
  Pos_BrakePedal[%]/1(Out1) -> Mux/2  "Pos_BrakePedal[%]"
  Pos_ClutchPedal[%]/1(Out1) -> Mux/3  "Pos_ClutchPedal[%]"
  Gear[]/1(Out1) -> Mux2/1  "Gear[]"
  Angle_SteeringWheel[deg]/1(Out1) -> DriverOverview/7  "Angle_SteeringWheel[deg]"
  SelectorLever[-3T|-2P|-1R|0N|1D]/1(Out1) -> Mux2/2  "SelectorLever[-3T|-2P|-1R|0N|1D]"
  v_Vehicle_Ref[km|h]/1(Out1) -> AbsoluteError/2(Set), RelativeError/2(Set), Mux1/2  "v_Vehicle_Ref[km|h]"
  e_Lat[m]/1(Out1) -> DriverOverview/8  "e_Lat[m]"
  Mux/1 -> DriverOverview/4
  Bus Selector1/1 -> v_x_Vehicle_CoG[km|h]/1(In1)  "<v_x_Vehicle_CoG[km|h]>"
  Velocities/1 -> Bus Selector1/1
  Bus Selector2/1 -> v_Vehicle_Ref[km|h]/1(In1)  "<v_Vehicle_Ref[km|h]>"
  v_x_Vehicle_CoG[km|h]/1(Out1) -> AbsoluteError/1(Current), RelativeError/1(Current), Mux1/1
  Mux1/1 -> DriverOverview/1
  AbsoluteError/1(AbsoluteError[km|h]) -> DriverOverview/3  "AbsoluteError[km|h]"
  RelativeError/1(RelativeError[%]) -> DriverOverview/2  "RelativError[%]"
  Bus Selector2/2 -> Pos_AccPedal[%]/1(In1)  "<Pos_AccPedal[%]>"
  Bus Selector2/3 -> Pos_BrakePedal[%]/1(In1)  "<Pos_BrakePedal[%]>"
  Bus Selector2/4 -> Pos_ClutchPedal[%]/1(In1)  "<Pos_ClutchPedal[%]>"
  Bus Selector2/5 -> Gear[]/1(In1)  "<Gear[]>"
  Bus Selector2/6 -> SelectorLever[-3T|-2P|-1R|0N|1D]/1(In1)  "<SelectorLever[-3T|-2P|-1R|0N|1D]>"
  Mux2/1 -> DriverOverview/5
  Bus Selector3/2 -> Angle_SteeringWheel[deg]/1(In1)  "<Angle_SteeringWheel[deg]>"
  Bus Selector3/3 -> e_Lat[m]/1(In1)  "<e_Lat[m]>"
  Bus Selector3/1 -> a_x_Vehicle_Ref[m|s2]/1(In1)  "<a_x_Vehicle_Ref[m|s2]>"
  a_x_Vehicle_Ref[m|s2]/1(Out1) -> DriverOverview/6  "a_x_Vehicle_Ref[m|s2]"

== system ASM_Traffic_V2X_Complete_Model_2/MDLUserInterface/Environment/MDL_DISP/Maneuver ==
  Maneuver : Inport
  Bus Selector2 : BusSelector  OutputSignals=ManeuverScheduler.Info.CurrentSegment[],ManeuverScheduler.Info.t_local[s],ManeuverScheduler.Info.s_local[m],ManeuverScheduler.Info.ManeuverTime[s],ManeuverScheduler.Info.ManeuverState[],ManeuverScheduler.ModeSignals.Road_Mode[1NoRoad|2Straight|3Circle|4Road]
  CurrentSegment[] : Subsystem
      mask Display: disp('')
  ManeuverInfo : Scope  NumInputPorts=6
  ManeuverState[] : Subsystem
      mask Display: disp('')
  ManeuverTime[s] : Subsystem
      mask Display: disp('')
  Road_Mode[1NoRoad|2Straight|3Circle|4Road] : Subsystem
      mask Display: disp('')
  s_local[m] : Subsystem
      mask Display: disp('')
  t_local[s] : Subsystem
      mask Display: disp('')
  wires:
  Maneuver/1 -> Bus Selector2/1
  Bus Selector2/1 -> CurrentSegment[]/1(In1)  "<CurrentSegment[]>"
  CurrentSegment[]/1(Out1) -> ManeuverInfo/1  "CurrentSegment[]"
  Bus Selector2/2 -> t_local[s]/1(In1)  "<t_local[s]>"
  t_local[s]/1(Out1) -> ManeuverInfo/2  "t_local[s]"
  Bus Selector2/3 -> s_local[m]/1(In1)  "<s_local[m]>"
  s_local[m]/1(Out1) -> ManeuverInfo/3  "s_local[m]"
  Bus Selector2/4 -> ManeuverTime[s]/1(In1)  "<ManeuverTime[s]>"
  ManeuverTime[s]/1(Out1) -> ManeuverInfo/4  "ManeuverTime[s]"
  Bus Selector2/5 -> ManeuverState[]/1(In1)  "<ManeuverState[]>"
  ManeuverState[]/1(Out1) -> ManeuverInfo/5  "ManeuverState[]"
  Bus Selector2/6 -> Road_Mode[1NoRoad|2Straight|3Circle|4Road]/1(In1)  "<Road_Mode[1NoRoad|2Straight|3Circle|4Road]>"
  Road_Mode[1NoRoad|2Straight|3Circle|4Road]/1(Out1) -> ManeuverInfo/6  "Road_Mode[1NoRoad|2Straight|3Circle|4Road]"

== system ASM_Traffic_V2X_Complete_Model_2/MDLUserInterface/Environment/MDL_DISP/Road ==
  Road : Inport
  Angle_Yaw_Veh_Road[deg] : Subsystem
      mask Display: disp('')
  BorderMode : Display
  Bus Selector1 : BusSelector  OutputSignals=LaneSensor_Dynamic.Parameters.Border_Mode[0Center|1Inner|2Outer],LaneSensor_Dynamic.Sensor_Output.CurrentLane.Common.LaneWidth[m],LaneSensor_Dynamic.Sensor_Output.CurrentLane.LeftSide.MarkerType_Left[],LaneSensor_Dynamic.Sensor_Output.CurrentLane.RightSide.MarkerType_Right[],LaneSensor_Dynamic.Sensor_Output.CurrentLane.LeftSide.Distance_Marker_Left[m],LaneSensor_Dynamic.Sensor_Output.CurrentLane.RightSide.Distance_Marker_Right[m],LaneSensor_Dynamic.Sensor_Output.Measurement_Points.Distance_MeasPnt_Marker_Left[m],LaneSensor_Dynamic.Sensor_Output.Measurement_Points.Distance_MeasPnt_Marker_Right[m],LaneSensor_Dynamic.Sensor_Output.Measurement_Points.Velocity_MeasPnt_Marker_Left[m|s],LaneSensor_Dynamic.Sensor_Output.Measurement_Points.Velocity_MeasPnt_Marker_Right[m|s]
  Bus Selector2 : BusSelector  OutputSignals=Road_ASMVeh.Curv_Veh_Road[1|m],Road_ASMVeh.Slope_Veh_Road[%],Road_ContactPoints.Fric_Coeff_CP[:][],Road_ContactPoints.Pos_z_CP[:][m],Road_ContactPoints.Sw_Tire_Parameter_Set_CP[:][1|2|3|4],Road_ASMVeh.s_Veh_Road[m],Road_ASMVeh.Pos_x_Ref_Veh_Road[m],Road_ASMVeh.Pos_y_Ref_Veh_Road[m],Road_ASMVeh.Angle_Yaw_Veh_Road[deg],Pos_Vehicle_GPS[Long;Lat][deg].Longitude[deg],Pos_Vehicle_GPS[Long;Lat][deg].Latitude[deg]
  Curv_Veh_Road[1|m] : Subsystem
      mask Display: disp('')
  Display : Display
  Distance_Marker_Left[m] : Subsystem
      mask Display: disp('')
  Distance_Marker_Right[m] : Subsystem
      mask Display: disp('')
  Distance_MeasPnt1_Marker_Left[m] : Subsystem
      mask Display: disp('')
  Distance_MeasPnt1_Marker_Right[m] : Subsystem
      mask Display: disp('')
  Distance_MeasPnt2_Marker_Left[m] : Subsystem
      mask Display: disp('')
  Distance_MeasPnt2_Marker_Right[m] : Subsystem
      mask Display: disp('')
  Fric_Coeff_CP[:][] : Subsystem
      mask Display: disp('')
  GPS_Latitude_Road[deg] : Subsystem
      mask Display: disp('')
  GPS_Longitude_Road[deg] : Subsystem
      mask Display: disp('')
  LaneSensorDynamic : Scope  NumInputPorts=5
  LaneSensorDynamic_MeasPnts : Scope  NumInputPorts=8
  LaneWidth[m] : Subsystem
      mask Display: disp('')
  MarkerType_Left[] : Subsystem
      mask Display: disp('')
  MarkerType_Right[] : Subsystem
      mask Display: disp('')
  Pos_x_Ref_Veh_Road[m] : Subsystem
      mask Display: disp('')
  Pos_y_Ref_Veh_Road[m] : Subsystem
      mask Display: disp('')
  Pos_z_CP[:][m] : Subsystem
      mask Display: disp('')
  RoadOverview : Scope  NumInputPorts=5
  RoadPositions : Scope  NumInputPorts=6
  Selector{,1,4..5} (4 alike) : Selector  IndexOptions=Index vector (dialog)  Indices=[1]  OutputSizes=1
  Selector{2..3,6..7} (4 alike) : Selector  IndexOptions=Index vector (dialog)  Indices=[2]  OutputSizes=1
  Slope_Veh_Road[%] : Subsystem
      mask Display: disp('')
  Sw_Tire_Parameter_Set_CP[:][1|2|3|4] : Subsystem
      mask Display: disp('')
  Velocity_MeasPnt1_Marker_Left[m|s] : Subsystem
      mask Display: disp('')
  Velocity_MeasPnt1_Marker_Right[m|s] : Subsystem
      mask Display: disp('')
  Velocity_MeasPnt2_Marker_Left[m|s] : Subsystem
      mask Display: disp('')
  Velocity_MeasPnt2_Marker_Right[m|s] : Subsystem
      mask Display: disp('')
  s_Veh_Road[m] : Subsystem
      mask Display: disp('')
  wires:
  Road/1 -> Bus Selector1/1, Bus Selector2/1
  Bus Selector2/1 -> Curv_Veh_Road[1|m]/1(In1)  "<Curv_Veh_Road[1|m]>"
  Curv_Veh_Road[1|m]/1(Out1) -> RoadOverview/1  "Curv_Veh_Road[1|m]"
  Bus Selector2/2 -> Slope_Veh_Road[%]/1(In1)  "<Slope_Veh_Road[%]>"
  Slope_Veh_Road[%]/1(Out1) -> RoadOverview/2  "Slope_Veh_Road[%]"
  Bus Selector2/3 -> Fric_Coeff_CP[:][]/1(In1)  "<Fric_Coeff_CP[:][]>"
  Fric_Coeff_CP[:][]/1(Out1) -> RoadOverview/3  "Fric_Coeff_CP[:][]"
  Bus Selector2/4 -> Pos_z_CP[:][m]/1(In1)  "<Pos_z_CP[:][m]>"
  Pos_z_CP[:][m]/1(Out1) -> RoadOverview/4  "Pos_z_CP[:][m]"
  Bus Selector2/5 -> Sw_Tire_Parameter_Set_CP[:][1|2|3|4]/1(In1)  "<Sw_Tire_Parameter_Set_CP[:][1|2|3|4]>"
  Sw_Tire_Parameter_Set_CP[:][1|2|3|4]/1(Out1) -> RoadOverview/5  "Sw_Tire_Parameter_Set_CP[:][1|2|3|4]"
  Bus Selector2/6 -> s_Veh_Road[m]/1(In1)  "<s_Veh_Road[m]>"
  s_Veh_Road[m]/1(Out1) -> Display/1, RoadPositions/1  "s_Veh_Road[m]"
  Bus Selector2/7 -> Pos_x_Ref_Veh_Road[m]/1(In1)  "<Pos_x_Ref_Veh_Road[m]>"
  Pos_x_Ref_Veh_Road[m]/1(Out1) -> RoadPositions/2  "Pos_x_Ref_Veh_Road[m]"
  Bus Selector2/8 -> Pos_y_Ref_Veh_Road[m]/1(In1)  "<Pos_y_Ref_Veh_Road[m]>"
  Pos_y_Ref_Veh_Road[m]/1(Out1) -> RoadPositions/3  "Pos_y_Ref_Veh_Road[m]"
  Bus Selector2/9 -> Angle_Yaw_Veh_Road[deg]/1(In1)  "<Angle_Yaw_Veh_Road[deg]>"
  Angle_Yaw_Veh_Road[deg]/1(Out1) -> RoadPositions/4  "Angle_Yaw_Veh_Road[deg]"
  Bus Selector2/11 -> GPS_Latitude_Road[deg]/1(In1)  "<Latitude[deg]>"
  Bus Selector2/10 -> GPS_Longitude_Road[deg]/1(In1)  "<Longitude[deg]>"
  GPS_Longitude_Road[deg]/1(Out1) -> RoadPositions/5  "GPS_Longitude_Road[deg]"
  GPS_Latitude_Road[deg]/1(Out1) -> RoadPositions/6  "GPS_Latitude_Road[deg]"
  Selector/1 -> Distance_MeasPnt1_Marker_Left[m]/1(In1)
  Selector4/1 -> Distance_MeasPnt1_Marker_Right[m]/1(In1)
  Selector1/1 -> Velocity_MeasPnt1_Marker_Left[m|s]/1(In1)
  Selector5/1 -> Velocity_MeasPnt1_Marker_Right[m|s]/1(In1)
  Selector2/1 -> Distance_MeasPnt2_Marker_Left[m]/1(In1)
  Selector6/1 -> Distance_MeasPnt2_Marker_Right[m]/1(In1)
  Selector3/1 -> Velocity_MeasPnt2_Marker_Left[m|s]/1(In1)
  Selector7/1 -> Velocity_MeasPnt2_Marker_Right[m|s]/1(In1)
  Distance_Marker_Right[m]/1(Out1) -> LaneSensorDynamic/5  "Distance_Marker_Right[m]"
  LaneWidth[m]/1(Out1) -> LaneSensorDynamic/1  "LaneWidth[m]"
  MarkerType_Left[]/1(Out1) -> LaneSensorDynamic/2  "MarkerType_Left[]"
  MarkerType_Right[]/1(Out1) -> LaneSensorDynamic/3  "MarkerType_Right[]"
  Distance_Marker_Left[m]/1(Out1) -> LaneSensorDynamic/4  "Distance_Marker_Left[m]"
  Distance_MeasPnt2_Marker_Left[m]/1(Out1) -> LaneSensorDynamic_MeasPnts/5  "Distance_MeasPnt2_Marker_Left[m]"
  Distance_MeasPnt2_Marker_Right[m]/1(Out1) -> LaneSensorDynamic_MeasPnts/6  "Distance_MeasPnt2_Marker_Right[m]"
  Velocity_MeasPnt2_Marker_Left[m|s]/1(Out1) -> LaneSensorDynamic_MeasPnts/7  "Velocity_MeasPnt2_Marker_Left[m|s]"
  Velocity_MeasPnt2_Marker_Right[m|s]/1(Out1) -> LaneSensorDynamic_MeasPnts/8  "Velocity_MeasPnt2_Marker_Right[m|s]"
  Distance_MeasPnt1_Marker_Left[m]/1(Out1) -> LaneSensorDynamic_MeasPnts/1  "Distance_MeasPnt1_Marker_Left[m]"
  Distance_MeasPnt1_Marker_Right[m]/1(Out1) -> LaneSensorDynamic_MeasPnts/2  "Distance_MeasPnt1_Marker_Right[m]"
  Velocity_MeasPnt1_Marker_Left[m|s]/1(Out1) -> LaneSensorDynamic_MeasPnts/3  "Velocity_MeasPnt1_Marker_Left[m|s]"
  Velocity_MeasPnt1_Marker_Right[m|s]/1(Out1) -> LaneSensorDynamic_MeasPnts/4  "Velocity_MeasPnt1_Marker_Right[m|s]"
  Bus Selector1/1 -> BorderMode/1  "<Border_Mode[0Center|1Inner|2Outer]>"
  Bus Selector1/2 -> LaneWidth[m]/1(In1)  "<LaneWidth[m]>"
  Bus Selector1/3 -> MarkerType_Left[]/1(In1)  "<MarkerType_Left[]>"
  Bus Selector1/4 -> MarkerType_Right[]/1(In1)  "<MarkerType_Right[]>"
  Bus Selector1/5 -> Distance_Marker_Left[m]/1(In1)  "<Distance_Marker_Left[m]>"
  Bus Selector1/6 -> Distance_Marker_Right[m]/1(In1)  "<Distance_Marker_Right[m]>"
  Bus Selector1/7 -> Selector2/1, Selector/1  "<Distance_MeasPnt_Marker_Left[m]>"
  Bus Selector1/8 -> Selector6/1, Selector4/1  "<Distance_MeasPnt_Marker_Right[m]>"
  Bus Selector1/9 -> Selector3/1, Selector1/1  "<Velocity_MeasPnt_Marker_Left[m|s]>"
  Bus Selector1/10 -> Selector7/1, Selector5/1  "<Velocity_MeasPnt_Marker_Right[m|s]>"

== system ASM_Traffic_V2X_Complete_Model_2/MDLUserInterface/Environment/MDL_DISP/Traffic ==
  ASMSignalBus : Inport
  Bus Selector5 : BusSelector  OutputSignals=FellowMovement.TrafficScheduler.Info.TrafficState[]
  Custom_Sensor : Subsystem
  Fellow_Movement : Subsystem
  Line_Sensor : Subsystem
  Object_Sensor_2D : Subsystem
  Object_Sensor_3D : Subsystem
  TrafficState[] : Subsystem
      mask Display: disp('')
  Traffic_Sign_Sensor : Subsystem
  Traffic_State : Scope
  wires:
  ASMSignalBus/1 -> Fellow_Movement/1(TrafficBus), Object_Sensor_3D/1(TrafficBus), Object_Sensor_2D/1(TrafficBus), Traffic_Sign_Sensor/1(TrafficBus), Line_Sensor/1(TrafficBus), Custom_Sensor/1(TrafficBus), Bus Selector5/1
  Bus Selector5/1 -> TrafficState[]/1(In1)  "<TrafficState[]>"
  TrafficState[]/1(Out1) -> Traffic_State/1  "TrafficState[]"

== system ASM_Traffic_V2X_Complete_Model_2/MDLUserInterface/Environment/MDL_PAR/BasicRoad ==
  Bus Creator : BusCreator  Inputs=4
  Fric_Coeff_BasicRoad[] : Constant
  Gain_Fric_Coeff_BasicRoad[FL;FR;RL;RR] : Gain  Gain=[1 1 1 1]
  Gain_Tire_Parameter_Set[FL;FR;RL;RR][1|2|3|4] : Gain  Gain=[1 1 1 1]
  Slope_BasicRoad[%] : Constant  Value=0
  Slope_Lateral_BasicRoad[deg] : Constant  Value=0
  Sw_Tire_Parameter_Set[1|2|3|4] : Constant
  tag scope: TAG_Sw_BasicRoad=global
  wires:
  Bus Creator/1 -> [TAG_Sw_BasicRoad]
  Slope_BasicRoad[%]/1 -> Bus Creator/1  "Slope_BasicRoad[%]"
  Slope_Lateral_BasicRoad[deg]/1 -> Bus Creator/2  "Slope_Lateral_BasicRoad[deg]"
  Fric_Coeff_BasicRoad[]/1 -> Gain_Fric_Coeff_BasicRoad[FL;FR;RL;RR]/1
  Gain_Fric_Coeff_BasicRoad[FL;FR;RL;RR]/1 -> Bus Creator/3  "Fric_Coeff_CP_BasicRoad[:][]"
  Sw_Tire_Parameter_Set[1|2|3|4]/1 -> Gain_Tire_Parameter_Set[FL;FR;RL;RR][1|2|3|4]/1
  Gain_Tire_Parameter_Set[FL;FR;RL;RR][1|2|3|4]/1 -> Bus Creator/4  "Sw_Tire_Parameter_Set_CP_BasicRoad[:][1|2|3|4]"

== system ASM_Traffic_V2X_Complete_Model_2/MDLUserInterface/Environment/MDL_PAR/CollisionSensor ==
  Bus Creator2 : BusCreator  Inputs=3
  Pos_x_CollisionObj_Custom_RefPnt[m] : Constant  Value=[0.02,-0.0555,-0.68, 0.89, 0.89]
  Pos_y_CollisionObj_Custom_RefPnt[m] : Constant  Value=[0.27,0.15,0.27,0.85,-0.85]
  TrafficObject_Type_CollisionObj[] : Constant  Value=[122,123,124,84,80]
  tag scope: TAG_CollisionSensor_Parameters=global
  wires:
  Bus Creator2/1 -> [TAG_CollisionSensor_Parameters]
  TrafficObject_Type_CollisionObj[]/1 -> Bus Creator2/1  "TrafficObject_Type_CollisionObj[]"
  Pos_y_CollisionObj_Custom_RefPnt[m]/1 -> Bus Creator2/3  "Pos_y_CollisionObj_Custom_RefPnt[m]"
  Pos_x_CollisionObj_Custom_RefPnt[m]/1 -> Bus Creator2/2  "Pos_x_CollisionObj_Custom_RefPnt[m]"
